simulink model "SystemSISOC"  (Simulink 6.3)
settings: Solver=ode45  StartTime=0.0  StopTime=tend  MaxStep=0.01  RelTol=1e-3
values from neighbouring files (symbols this model uses):
  Tp = 0.1    [zad_1_1.m]    (also in zad_1_2.m; zad_2_RIV.m; zad_2_RLS.m)
undefined symbols (not defined in the file or in its folder): sigma2e
libraries: simulink x1
settings Model: LastModifiedBy=Maciej

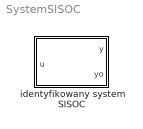
== system SystemSISOC ==
  identyfikowany system SISOC : Subsystem

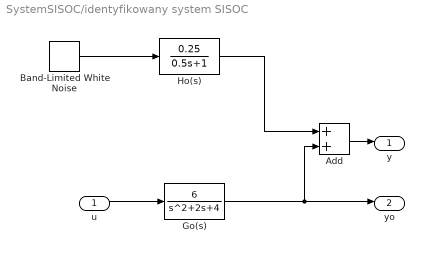
== system SystemSISOC/identyfikowany system SISOC ==
  u : Inport
  Add : Sum  OutScaling=2^-10
  Band-Limited White Noise : simulink/Sources/Band-Limited White Noise  Cov=[sigma2e]  Ts=Tp*0.1  seed=[2941]
  Go(s) : TransferFcn  Numerator=[6]  Denominator=[1 2 4]
  Ho(s) : TransferFcn  Numerator=[0.25]  Denominator=[0.5 1]
  y : Outport
  yo : Outport  Port=2
  wires:
  Band-Limited White Noise/1 -> Ho(s)/1
  Ho(s)/1 -> Add/1
  Go(s)/1 -> Add/2, yo/1
  Add/1 -> y/1
  u/1 -> Go(s)/1
